simulink library "halin"  (R2021b)
settings: Solver=VariableStepAuto  StartTime=0.0  StopTime=10.0  RelTol=1e-3
undefined symbols (not defined in the file): TRUE
libraries: FVT_lib x177, hcu_lib x55
(part 5 of 17)

== system halin/HAL_IN/CAN5 ==
  DT_CAN5_SG_TBOX1 : Inport
  DT_CAN5_SG_TBOX2 : Inport  Port=2
  DT_CAN5_SG_TBOX3 : Inport  Port=3
  TBOX1 : Subsystem
  TBOX2 : Subsystem
  TBOX3 : Subsystem
  UnitConverter{,2,4,8..10} (6 alike) : DataTypeConversion  OutDataTypeStr=uint8
  UnitConverter{1,6,11..27} (19 alike) : DataTypeConversion  OutDataTypeStr=single
  UnitConverter28 : DataTypeConversion  OutDataTypeStr=uint32
  UnitConverter29 : DataTypeConversion  OutDataTypeStr=uint32
  UnitConverter3 : DataTypeConversion  OutDataTypeStr=uint16
  UnitConverter5 : DataTypeConversion  OutDataTypeStr=boolean
  UnitConverter7 : DataTypeConversion  OutDataTypeStr=boolean
  VHAL_CANMsgInvalidTBOX1_flg : Subsystem  AncestorBlock=FVT_lib/hal/MsgTimeoutJudge_CAN_AUTOSAR
      mask help: MeasumentTrigerEvent
      mask Display: fprintf('MsgTimeoutJudge_CAN\nAUTOSAR');
  VHAL_CANMsgInvalidTBOX2_flg : Subsystem  AncestorBlock=FVT_lib/hal/MsgTimeoutJudge_CAN_AUTOSAR
      mask help: MeasumentTrigerEvent
      mask Display: fprintf('MsgTimeoutJudge_CAN\nAUTOSAR');
  VHAL_CANMsgInvalidTBOX3_flg : Subsystem  AncestorBlock=FVT_lib/hal/MsgTimeoutJudge_CAN_AUTOSAR
      mask help: MeasumentTrigerEvent
      mask Display: fprintf('MsgTimeoutJudge_CAN\nAUTOSAR');
  bus_creator : BusCreator  Inputs=33
  HAL_CAN5_outputs : Outport
  wires:
  DT_CAN5_SG_TBOX1/1 -> [DT_CAN5_SG_TBOX1]
  DT_CAN5_SG_TBOX2/1 -> [DT_CAN5_SG_TBOX2]
  DT_CAN5_SG_TBOX3/1 -> [DT_CAN5_SG_TBOX3]
  [DT_CAN5_SG_TBOX1] -> TBOX1/1(DT_CAN5_SG_TBOX1)
  [DT_CAN5_SG_TBOX2] -> TBOX2/1(DT_CAN5_SG_TBOX2)
  [DT_CAN5_SG_TBOX3] -> TBOX3/1(DT_CAN5_SG_TBOX3)
  bus_creator/1 -> HAL_CAN5_outputs/1
  VHAL_CANMsgInvalidTBOX1_flg/1(Out) -> bus_creator/1
  TBOX1/1(VHAL_CbnPreACEnaReq_enum) -> [VHAL_CbnPreACEnaReq_enum]
  UnitConverter/1 -> bus_creator/2  "VHAL_CbnPreACEnaReq_enum"
  [VHAL_CbnPreACEnaReq_enum] -> UnitConverter/1
  TBOX1/2(VHAL_PowerOffTSet_cnt) -> [VHAL_PowerOffTSet_cnt]
  UnitConverter1/1 -> bus_creator/3  "VHAL_PowerOffTSet_cnt"
  [VHAL_PowerOffTSet_cnt] -> UnitConverter1/1
  TBOX1/3(VHAL_ReOutsideMirror_enum) -> [VHAL_ReOutsideMirror_enum]
  UnitConverter2/1 -> bus_creator/4  "VHAL_ReOutsideMirror_enum"
  [VHAL_ReOutsideMirror_enum] -> UnitConverter2/1
  TBOX1/4(VHAL_ReDoorLock_enum) -> [VHAL_ReDoorLock_enum]
  UnitConverter3/1 -> bus_creator/5  "VHAL_ReDoorLock_enum"
  [VHAL_ReDoorLock_enum] -> UnitConverter3/1
  TBOX1/5(VHAL_RePwrReqTbox_enum) -> [VHAL_RePwrReqTbox_enum]
  UnitConverter4/1 -> bus_creator/6  "VHAL_RePwrReqTbox_enum"
  [VHAL_RePwrReqTbox_enum] -> UnitConverter4/1
  TBOX1/6(VHAL_ReRadio_flg) -> [VHAL_ReRadio_flg]
  UnitConverter5/1 -> bus_creator/7  "VHAL_ReRadio_flg"
  [VHAL_ReRadio_flg] -> UnitConverter5/1
  TBOX1/7(VHAL_RemoteACTemp_C) -> [VHAL_RemoteACTemp_C]
  UnitConverter6/1 -> bus_creator/8  "VHAL_RemoteACTemp_C"
  [VHAL_RemoteACTemp_C] -> UnitConverter6/1
  TBOX1/8(VHAL_RemoteAutoReq_flg) -> [VHAL_RemoteAutoReq_flg]
  UnitConverter7/1 -> bus_creator/9  "VHAL_RemoteAutoReq_flg"
  [VHAL_RemoteAutoReq_flg] -> UnitConverter7/1
  TBOX1/9(VHAL_TBOXNETSIGSTR_enum) -> [VHAL_TBOXNETSIGSTR_enum]
  UnitConverter8/1 -> bus_creator/10  "VHAL_TBOXNETSIGSTR_enum"
  [VHAL_TBOXNETSIGSTR_enum] -> UnitConverter8/1
  TBOX1/10(VHAL_TBOXRemotePW_enum) -> [VHAL_TBOXRemotePW_enum]
  UnitConverter9/1 -> bus_creator/11  "VHAL_TBOXRemotePW_enum"
  [VHAL_TBOXRemotePW_enum] -> UnitConverter9/1
  TBOX1/11(VHAL_TBOXTESTSTATUS_enum) -> [VHAL_TBOXTESTSTATUS_enum]
  UnitConverter10/1 -> bus_creator/12  "VHAL_TBOXTESTSTATUS_enum"
  [VHAL_TBOXTESTSTATUS_enum] -> UnitConverter10/1
  VHAL_CANMsgInvalidTBOX2_flg/1(Out) -> bus_creator/13
  TBOX2/1(VHAL_TimeSyncFromBSDay_DAY) -> [VHAL_TimeSyncFromBSDay_DAY]
  UnitConverter11/1 -> bus_creator/14  "VHAL_TimeSyncFromBSDay_DAY"
  [VHAL_TimeSyncFromBSDay_DAY] -> UnitConverter11/1
  TBOX2/2(VHAL_TimeSyncFromBSHour_hr) -> [VHAL_TimeSyncFromBSHour_hr]
  UnitConverter12/1 -> bus_creator/15  "VHAL_TimeSyncFromBSHour_hr"
  [VHAL_TimeSyncFromBSHour_hr] -> UnitConverter12/1
  TBOX2/3(VHAL_TimeSyncFromBSMinute_min) -> [VHAL_TimeSyncFromBSMinute_min]
  UnitConverter13/1 -> bus_creator/16  "VHAL_TimeSyncFromBSMinute_min"
  [VHAL_TimeSyncFromBSMinute_min] -> UnitConverter13/1
  TBOX2/4(VHAL_TimeSyncFromBSMonth_MONTH) -> [VHAL_TimeSyncFromBSMonth_MONTH]
  UnitConverter14/1 -> bus_creator/17  "VHAL_TimeSyncFromBSMonth_MONTH"
  [VHAL_TimeSyncFromBSMonth_MONTH] -> UnitConverter14/1
  TBOX2/5(VHAL_TimeSyncFromBSSecond_s) -> [VHAL_TimeSyncFromBSSecond_s]
  UnitConverter15/1 -> bus_creator/18  "VHAL_TimeSyncFromBSSecond_s"
  [VHAL_TimeSyncFromBSSecond_s] -> UnitConverter15/1
  TBOX2/6(VHAL_TimeSyncFromBSYear_YEAR) -> [VHAL_TimeSyncFromBSYear_YEAR]
  UnitConverter16/1 -> bus_creator/19  "VHAL_TimeSyncFromBSYear_YEAR"
  [VHAL_TimeSyncFromBSYear_YEAR] -> UnitConverter16/1
  VHAL_CANMsgInvalidTBOX3_flg/1(Out) -> bus_creator/20
  TBOX3/1(VHAL_ChargePercentSet_pct) -> [VHAL_ChargePercentSet_pct]
  UnitConverter17/1 -> bus_creator/21  "VHAL_ChargePercentSet_pct"
  [VHAL_ChargePercentSet_pct] -> UnitConverter17/1
  TBOX3/2(VHAL_ReserveChargeOFFDay_DAY) -> [VHAL_ReserveChargeOFFDay_DAY]
  UnitConverter18/1 -> bus_creator/22  "VHAL_ReserveChargeOFFDay_DAY"
  [VHAL_ReserveChargeOFFDay_DAY] -> UnitConverter18/1
  TBOX3/3(VHAL_ReserveChargeOFFHour_hr) -> [VHAL_ReserveChargeOFFHour_hr]
  UnitConverter19/1 -> bus_creator/23  "VHAL_ReserveChargeOFFHour_hr"
  [VHAL_ReserveChargeOFFHour_hr] -> UnitConverter19/1
  TBOX3/4(VHAL_ReserveChargeOFFMinute_min) -> [VHAL_ReserveChargeOFFMinute_min]
  UnitConverter20/1 -> bus_creator/24  "VHAL_ReserveChargeOFFMinute_min"
  [VHAL_ReserveChargeOFFMinute_min] -> UnitConverter20/1
  TBOX3/5(VHAL_ReserveChargeOFFMonth_MONTH) -> [VHAL_ReserveChargeOFFMonth_MONTH]
  UnitConverter21/1 -> bus_creator/25  "VHAL_ReserveChargeOFFMonth_MONTH"
  [VHAL_ReserveChargeOFFMonth_MONTH] -> UnitConverter21/1
  TBOX3/6(VHAL_ReserveChargeOFFYear_YEAR) -> [VHAL_ReserveChargeOFFYear_YEAR]
  UnitConverter22/1 -> bus_creator/26  "VHAL_ReserveChargeOFFYear_YEAR"
  [VHAL_ReserveChargeOFFYear_YEAR] -> UnitConverter22/1
  TBOX3/7(VHAL_ReserveChargeOnDay_DAY) -> [VHAL_ReserveChargeOnDay_DAY]
  UnitConverter23/1 -> bus_creator/27  "VHAL_ReserveChargeOnDay_DAY"
  [VHAL_ReserveChargeOnDay_DAY] -> UnitConverter23/1
  TBOX3/8(VHAL_ReserveChargeOnHour_hr) -> [VHAL_ReserveChargeOnHour_hr]
  UnitConverter24/1 -> bus_creator/28  "VHAL_ReserveChargeOnHour_hr"
  [VHAL_ReserveChargeOnHour_hr] -> UnitConverter24/1
  TBOX3/9(VHAL_ReserveChargeOnMinute_min) -> [VHAL_ReserveChargeOnMinute_min]
  UnitConverter25/1 -> bus_creator/29  "VHAL_ReserveChargeOnMinute_min"
  [VHAL_ReserveChargeOnMinute_min] -> UnitConverter25/1
  TBOX3/10(VHAL_ReserveChargeOnMonth_MONTH) -> [VHAL_ReserveChargeOnMonth_MONTH]
  UnitConverter26/1 -> bus_creator/30  "VHAL_ReserveChargeOnMonth_MONTH"
  [VHAL_ReserveChargeOnMonth_MONTH] -> UnitConverter26/1
  TBOX3/11(VHAL_ReserveChargeOnYear_YEAR) -> [VHAL_ReserveChargeOnYear_YEAR]
  UnitConverter27/1 -> bus_creator/31  "VHAL_ReserveChargeOnYear_YEAR"
  [VHAL_ReserveChargeOnYear_YEAR] -> UnitConverter27/1
  TBOX3/12(VHAL_TBOXHWVER_enum) -> [VHAL_TBOXHWVER_enum]
  UnitConverter28/1 -> bus_creator/32  "VHAL_TBOXHWVER_enum"
  [VHAL_TBOXHWVER_enum] -> UnitConverter28/1
  TBOX3/13(VHAL_TBOXSWVER_enum) -> [VHAL_TBOXSWVER_enum]
  UnitConverter29/1 -> bus_creator/33  "VHAL_TBOXSWVER_enum"
  [VHAL_TBOXSWVER_enum] -> UnitConverter29/1

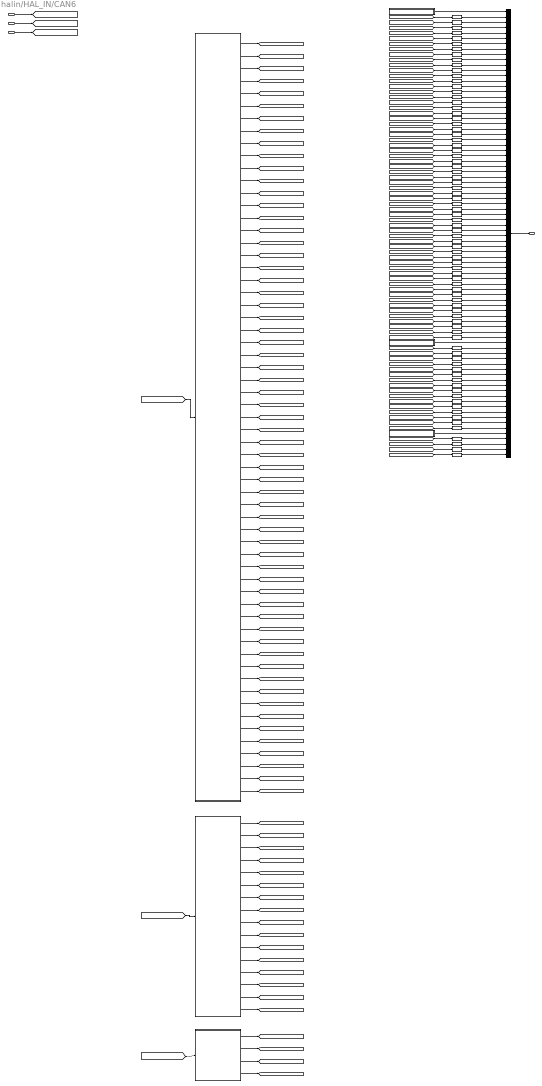
== system halin/HAL_IN/CAN6 ==
  DT_CAN6_SG_FCM1 : Inport
  DT_CAN6_SG_FCM3 : Inport  Port=2
  DT_CAN6_SG_SRR1 : Inport  Port=3
  FCM1 : Subsystem
  FCM3 : Subsystem
  SRR1 : Subsystem
  UnitConverter{,1..4,6..7,29..30,44,61..76} (26 alike) : DataTypeConversion  OutDataTypeStr=single
  UnitConverter{5,10..14,16,20,22..28,31..35,37..38,41..43,45,47,49,55,59..60,77..80} (35 alike) : DataTypeConversion  OutDataTypeStr=uint8
  UnitConverter{8..9,15,17..19,21,36,39..40,46,48,50..54,56..58} (20 alike) : DataTypeConversion  OutDataTypeStr=boolean
  VHAL_CANMsgInvalidFCM1_flg : Subsystem  AncestorBlock=FVT_lib/hal/MsgTimeoutJudge_CAN_AUTOSAR
      mask help: MeasumentTrigerEvent
      mask Display: fprintf('MsgTimeoutJudge_CAN\nAUTOSAR');
  VHAL_CANMsgInvalidFCM3_flg : Subsystem  AncestorBlock=FVT_lib/hal/MsgTimeoutJudge_CAN_AUTOSAR
      mask help: MeasumentTrigerEvent
      mask Display: fprintf('MsgTimeoutJudge_CAN\nAUTOSAR');
  VHAL_CANMsgInvalidSRR1_flg : Subsystem  AncestorBlock=FVT_lib/hal/MsgTimeoutJudge_CAN_AUTOSAR
      mask help: MeasumentTrigerEvent
      mask Display: fprintf('MsgTimeoutJudge_CAN\nAUTOSAR');
  bus_creator : BusCreator  Inputs=84
  HAL_CAN6_outputs : Outport
  wires:
  DT_CAN6_SG_FCM1/1 -> [DT_CAN6_SG_FCM1]
  DT_CAN6_SG_FCM3/1 -> [DT_CAN6_SG_FCM3]
  DT_CAN6_SG_SRR1/1 -> [DT_CAN6_SG_SRR1]
  [DT_CAN6_SG_FCM1] -> FCM1/1(DT_CAN6_SG_FCM1)
  [DT_CAN6_SG_FCM3] -> FCM3/1(DT_CAN6_SG_FCM3)
  [DT_CAN6_SG_SRR1] -> SRR1/1(DT_CAN6_SG_SRR1)
  bus_creator/1 -> HAL_CAN6_outputs/1
  VHAL_CANMsgInvalidFCM1_flg/1(Out) -> bus_creator/1
  FCM1/1(VHAL_ACCComfortBandLower_mps2) -> [VHAL_ACCComfortBandLower_mps2]
  UnitConverter/1 -> bus_creator/2  "VHAL_ACCComfortBandLower_mps2"
  [VHAL_ACCComfortBandLower_mps2] -> UnitConverter/1
  FCM1/2(VHAL_ACCComfortBandUpper_mps2) -> [VHAL_ACCComfortBandUpper_mps2]
  UnitConverter1/1 -> bus_creator/3  "VHAL_ACCComfortBandUpper_mps2"
  [VHAL_ACCComfortBandUpper_mps2] -> UnitConverter1/1
  FCM1/3(VHAL_ACCJerkLowerLimit_mps3) -> [VHAL_ACCJerkLowerLimit_mps3]
  UnitConverter2/1 -> bus_creator/4  "VHAL_ACCJerkLowerLimit_mps3"
  [VHAL_ACCJerkLowerLimit_mps3] -> UnitConverter2/1
  FCM1/4(VHAL_ACCJerkUpperLimit_mps3) -> [VHAL_ACCJerkUpperLimit_mps3]
  UnitConverter3/1 -> bus_creator/5  "VHAL_ACCJerkUpperLimit_mps3"
  [VHAL_ACCJerkUpperLimit_mps3] -> UnitConverter3/1
  FCM1/5(VHAL_ACCObjDist_m) -> [VHAL_ACCObjDist_m]
  UnitConverter4/1 -> bus_creator/6  "VHAL_ACCObjDist_m"
  [VHAL_ACCObjDist_m] -> UnitConverter4/1
  FCM1/6(VHAL_ACCObjDstLvl_enum) -> [VHAL_ACCObjDstLvl_enum]
  UnitConverter5/1 -> bus_creator/7  "VHAL_ACCObjDstLvl_enum"
  [VHAL_ACCObjDstLvl_enum] -> UnitConverter5/1
  FCM1/7(VHAL_ACCObjRelSpd_mps) -> [VHAL_ACCObjRelSpd_mps]
  UnitConverter6/1 -> bus_creator/8  "VHAL_ACCObjRelSpd_mps"
  [VHAL_ACCObjRelSpd_mps] -> UnitConverter6/1
  FCM1/8(VHAL_ACCRequiredAccel_mps2) -> [VHAL_ACCRequiredAccel_mps2]
  UnitConverter7/1 -> bus_creator/9  "VHAL_ACCRequiredAccel_mps2"
  [VHAL_ACCRequiredAccel_mps2] -> UnitConverter7/1
  FCM1/9(VHAL_ACCTakeoverReq_flg) -> [VHAL_ACCTakeoverReq_flg]
  UnitConverter8/1 -> bus_creator/10  "VHAL_ACCTakeoverReq_flg"
  [VHAL_ACCTakeoverReq_flg] -> UnitConverter8/1
  FCM1/10(VHAL_ACCVehHoldReq_flg) -> [VHAL_ACCVehHoldReq_flg]
  UnitConverter9/1 -> bus_creator/11  "VHAL_ACCVehHoldReq_flg"
  [VHAL_ACCVehHoldReq_flg] -> UnitConverter9/1
  FCM1/11(VHAL_ADASACCSta_enum) -> [VHAL_ADASACCSta_enum]
  UnitConverter10/1 -> bus_creator/12  "VHAL_ADASACCSta_enum"
  [VHAL_ADASACCSta_enum] -> UnitConverter10/1
  FCM1/12(VHAL_ADASAEBReq_enum) -> [VHAL_ADASAEBReq_enum]
  UnitConverter11/1 -> bus_creator/13  "VHAL_ADASAEBReq_enum"
  [VHAL_ADASAEBReq_enum] -> UnitConverter11/1
  FCM1/13(VHAL_ADASAEBSta_enum) -> [VHAL_ADASAEBSta_enum]
  UnitConverter12/1 -> bus_creator/14  "VHAL_ADASAEBSta_enum"
  [VHAL_ADASAEBSta_enum] -> UnitConverter12/1
  FCM1/14(VHAL_ADASCAMSpdLim_enum) -> [VHAL_ADASCAMSpdLim_enum]
  UnitConverter13/1 -> bus_creator/15  "VHAL_ADASCAMSpdLim_enum"
  [VHAL_ADASCAMSpdLim_enum] -> UnitConverter13/1
  FCM1/15(VHAL_ADASDBSReq_enum) -> [VHAL_ADASDBSReq_enum]
  UnitConverter14/1 -> bus_creator/16  "VHAL_ADASDBSReq_enum"
  [VHAL_ADASDBSReq_enum] -> UnitConverter14/1
  FCM1/16(VHAL_ADASFCWMute_flg) -> [VHAL_ADASFCWMute_flg]
  UnitConverter15/1 -> bus_creator/17  "VHAL_ADASFCWMute_flg"
  [VHAL_ADASFCWMute_flg] -> UnitConverter15/1
  FCM1/17(VHAL_ADASFCWSta_enum) -> [VHAL_ADASFCWSta_enum]
  UnitConverter16/1 -> bus_creator/18  "VHAL_ADASFCWSta_enum"
  [VHAL_ADASFCWSta_enum] -> UnitConverter16/1
  FCM1/18(VHAL_ADASFaultSta_flg) -> [VHAL_ADASFaultSta_flg]
  UnitConverter17/1 -> bus_creator/19  "VHAL_ADASFaultSta_flg"
  [VHAL_ADASFaultSta_flg] -> UnitConverter17/1
  FCM1/19(VHAL_ADASFltWrnReq_flg) -> [VHAL_ADASFltWrnReq_flg]
  UnitConverter18/1 -> bus_creator/20  "VHAL_ADASFltWrnReq_flg"
  [VHAL_ADASFltWrnReq_flg] -> UnitConverter18/1
  FCM1/20(VHAL_ADASForceIdle_flg) -> [VHAL_ADASForceIdle_flg]
  UnitConverter19/1 -> bus_creator/21  "VHAL_ADASForceIdle_flg"
  [VHAL_ADASForceIdle_flg] -> UnitConverter19/1
  FCM1/21(VHAL_ADASISASta_enum) -> [VHAL_ADASISASta_enum]
  UnitConverter20/1 -> bus_creator/22  "VHAL_ADASISASta_enum"
  [VHAL_ADASISASta_enum] -> UnitConverter20/1
  FCM1/22(VHAL_ADASLDWMute_flg) -> [VHAL_ADASLDWMute_flg]
  UnitConverter21/1 -> bus_creator/23  "VHAL_ADASLDWMute_flg"
  [VHAL_ADASLDWMute_flg] -> UnitConverter21/1
  FCM1/23(VHAL_ADASLDWSta_enum) -> [VHAL_ADASLDWSta_enum]
  UnitConverter22/1 -> bus_creator/24  "VHAL_ADASLDWSta_enum"
  [VHAL_ADASLDWSta_enum] -> UnitConverter22/1
  FCM1/24(VHAL_ADASLFCHandsOffWarning_enum) -> [VHAL_ADASLFCHandsOffWarning_enum]
  UnitConverter23/1 -> bus_creator/25  "VHAL_ADASLFCHandsOffWarning_enum"
  [VHAL_ADASLFCHandsOffWarning_enum] -> UnitConverter23/1
  FCM1/25(VHAL_ADASLFCSta_enum) -> [VHAL_ADASLFCSta_enum]
  UnitConverter24/1 -> bus_creator/26  "VHAL_ADASLFCSta_enum"
  [VHAL_ADASLFCSta_enum] -> UnitConverter24/1
  FCM1/26(VHAL_ADASLFCWarnSound_enum) -> [VHAL_ADASLFCWarnSound_enum]
  UnitConverter25/1 -> bus_creator/27  "VHAL_ADASLFCWarnSound_enum"
  [VHAL_ADASLFCWarnSound_enum] -> UnitConverter25/1
  FCM1/27(VHAL_ADASLKASta_enum) -> [VHAL_ADASLKASta_enum]
  UnitConverter26/1 -> bus_creator/28  "VHAL_ADASLKASta_enum"
  [VHAL_ADASLKASta_enum] -> UnitConverter26/1
  FCM1/28(VHAL_ADASLaneModeL_enum) -> [VHAL_ADASLaneModeL_enum]
  UnitConverter27/1 -> bus_creator/29  "VHAL_ADASLaneModeL_enum"
  [VHAL_ADASLaneModeL_enum] -> UnitConverter27/1
  FCM1/29(VHAL_ADASLaneModeR_enum) -> [VHAL_ADASLaneModeR_enum]
  UnitConverter28/1 -> bus_creator/30  "VHAL_ADASLaneModeR_enum"
  [VHAL_ADASLaneModeR_enum] -> UnitConverter28/1
  FCM1/30(VHAL_ADASLanecurveL_raw32) -> [VHAL_ADASLanecurveL_raw32]
  UnitConverter29/1 -> bus_creator/31  "VHAL_ADASLanecurveL_raw32"
  [VHAL_ADASLanecurveL_raw32] -> UnitConverter29/1
  FCM1/31(VHAL_ADASLanecurveR_raw32) -> [VHAL_ADASLanecurveR_raw32]
  UnitConverter30/1 -> bus_creator/32  "VHAL_ADASLanecurveR_raw32"
  [VHAL_ADASLanecurveR_raw32] -> UnitConverter30/1
  FCM1/32(VHAL_ADASLanetypeL_enum) -> [VHAL_ADASLanetypeL_enum]
  UnitConverter31/1 -> bus_creator/33  "VHAL_ADASLanetypeL_enum"
  [VHAL_ADASLanetypeL_enum] -> UnitConverter31/1
  FCM1/33(VHAL_ADASLanetypeR_enum) -> [VHAL_ADASLanetypeR_enum]
  UnitConverter32/1 -> bus_creator/34  "VHAL_ADASLanetypeR_enum"
  [VHAL_ADASLanetypeR_enum] -> UnitConverter32/1
  FCM1/34(VHAL_ADASSLIFSpdLim_enum) -> [VHAL_ADASSLIFSpdLim_enum]
  UnitConverter33/1 -> bus_creator/35  "VHAL_ADASSLIFSpdLim_enum"
  [VHAL_ADASSLIFSpdLim_enum] -> UnitConverter33/1
  FCM1/35(VHAL_ADASSLIFSta_enum) -> [VHAL_ADASSLIFSta_enum]
  UnitConverter34/1 -> bus_creator/36  "VHAL_ADASSLIFSta_enum"
  [VHAL_ADASSLIFSta_enum] -> UnitConverter34/1
  FCM1/36(VHAL_ADASShftPosnReq_enum) -> [VHAL_ADASShftPosnReq_enum]
  UnitConverter35/1 -> bus_creator/37  "VHAL_ADASShftPosnReq_enum"
  [VHAL_ADASShftPosnReq_enum] -> UnitConverter35/1
  FCM1/37(VHAL_ADASShftPosnReqA_flg) -> [VHAL_ADASShftPosnReqA_flg]
  UnitConverter36/1 -> bus_creator/38  "VHAL_ADASShftPosnReqA_flg"
  [VHAL_ADASShftPosnReqA_flg] -> UnitConverter36/1
  FCM1/38(VHAL_ADASVehSpdLim_enum) -> [VHAL_ADASVehSpdLim_enum]
  UnitConverter37/1 -> bus_creator/39  "VHAL_ADASVehSpdLim_enum"
  [VHAL_ADASVehSpdLim_enum] -> UnitConverter37/1
  FCM1/39(VHAL_ADASWarningMsg_enum) -> [VHAL_ADASWarningMsg_enum]
  UnitConverter38/1 -> bus_creator/40  "VHAL_ADASWarningMsg_enum"
  [VHAL_ADASWarningMsg_enum] -> UnitConverter38/1
  FCM1/40(VHAL_AEBVehHoldReq_flg) -> [VHAL_AEBVehHoldReq_flg]
  UnitConverter39/1 -> bus_creator/41  "VHAL_AEBVehHoldReq_flg"
  [VHAL_AEBVehHoldReq_flg] -> UnitConverter39/1
  FCM1/41(VHAL_CameraBlockage_flg) -> [VHAL_CameraBlockage_flg]
  UnitConverter40/1 -> bus_creator/42  "VHAL_CameraBlockage_flg"
  [VHAL_CameraBlockage_flg] -> UnitConverter40/1
  FCM1/42(VHAL_FCM1Checksum_enum) -> [VHAL_FCM1Checksum_enum]
  UnitConverter41/1 -> bus_creator/43  "VHAL_FCM1Checksum_enum"
  [VHAL_FCM1Checksum_enum] -> UnitConverter41/1
  FCM1/43(VHAL_FCM1LifeCount_enum) -> [VHAL_FCM1LifeCount_enum]
  UnitConverter42/1 -> bus_creator/44  "VHAL_FCM1LifeCount_enum"
  [VHAL_FCM1LifeCount_enum] -> UnitConverter42/1
  FCM1/44(VHAL_FCMACCmode_enum) -> [VHAL_FCMACCmode_enum]
  UnitConverter43/1 -> bus_creator/45  "VHAL_FCMACCmode_enum"
  [VHAL_FCMACCmode_enum] -> UnitConverter43/1
  FCM1/45(VHAL_FCMLKAStrToqReq_Nm) -> [VHAL_FCMLKAStrToqReq_Nm]
  UnitConverter44/1 -> bus_creator/46  "VHAL_FCMLKAStrToqReq_Nm"
  [VHAL_FCMLKAStrToqReq_Nm] -> UnitConverter44/1
  FCM1/46(VHAL_FCMLKATOIAct_enum) -> [VHAL_FCMLKATOIAct_enum]
  UnitConverter45/1 -> bus_creator/47  "VHAL_FCMLKATOIAct_enum"
  [VHAL_FCMLKATOIAct_enum] -> UnitConverter45/1
  FCM1/47(VHAL_FCMLKATOIFault_flg) -> [VHAL_FCMLKATOIFault_flg]
  UnitConverter46/1 -> bus_creator/48  "VHAL_FCMLKATOIFault_flg"
  [VHAL_FCMLKATOIFault_flg] -> UnitConverter46/1
  FCM1/48(VHAL_ForceLowBeam_enum) -> [VHAL_ForceLowBeam_enum]
  UnitConverter47/1 -> bus_creator/49  "VHAL_ForceLowBeam_enum"
  [VHAL_ForceLowBeam_enum] -> UnitConverter47/1
  FCM1/49(VHAL_HazardWarningReq_flg) -> [VHAL_HazardWarningReq_flg]
  UnitConverter48/1 -> bus_creator/50  "VHAL_HazardWarningReq_flg"
  [VHAL_HazardWarningReq_flg] -> UnitConverter48/1
  FCM1/50(VHAL_ISAWarningMsg_enum) -> [VHAL_ISAWarningMsg_enum]
  UnitConverter49/1 -> bus_creator/51  "VHAL_ISAWarningMsg_enum"
  [VHAL_ISAWarningMsg_enum] -> UnitConverter49/1
  FCM1/51(VHAL_LKAHODDisplayWarning_flg) -> [VHAL_LKAHODDisplayWarning_flg]
  UnitConverter50/1 -> bus_creator/52  "VHAL_LKAHODDisplayWarning_flg"
  [VHAL_LKAHODDisplayWarning_flg] -> UnitConverter50/1
  FCM1/52(VHAL_LKAHODSoundWarning_flg) -> [VHAL_LKAHODSoundWarning_flg]
  UnitConverter51/1 -> bus_creator/53  "VHAL_LKAHODSoundWarning_flg"
  [VHAL_LKAHODSoundWarning_flg] -> UnitConverter51/1
  FCM1/53(VHAL_LVDAACCStatusInformation_flg) -> [VHAL_LVDAACCStatusInformation_flg]
  UnitConverter52/1 -> bus_creator/54  "VHAL_LVDAACCStatusInformation_flg"
  [VHAL_LVDAACCStatusInformation_flg] -> UnitConverter52/1
  FCM1/54(VHAL_LVDADisabled_flg) -> [VHAL_LVDADisabled_flg]
  UnitConverter53/1 -> bus_creator/55  "VHAL_LVDADisabled_flg"
  [VHAL_LVDADisabled_flg] -> UnitConverter53/1
  FCM1/55(VHAL_LVDAFailinfo_flg) -> [VHAL_LVDAFailinfo_flg]
  UnitConverter54/1 -> bus_creator/56  "VHAL_LVDAFailinfo_flg"
  [VHAL_LVDAFailinfo_flg] -> UnitConverter54/1
  FCM1/56(VHAL_LVDAMuteSta_enum) -> [VHAL_LVDAMuteSta_enum]
  UnitConverter55/1 -> bus_creator/57  "VHAL_LVDAMuteSta_enum"
  [VHAL_LVDAMuteSta_enum] -> UnitConverter55/1
  FCM1/57(VHAL_LVDAWarning_flg) -> [VHAL_LVDAWarning_flg]
  UnitConverter56/1 -> bus_creator/58  "VHAL_LVDAWarning_flg"
  [VHAL_LVDAWarning_flg] -> UnitConverter56/1
  FCM1/58(VHAL_LeftTurnLightReq_flg) -> [VHAL_LeftTurnLightReq_flg]
  UnitConverter57/1 -> bus_creator/59  "VHAL_LeftTurnLightReq_flg"
  [VHAL_LeftTurnLightReq_flg] -> UnitConverter57/1
  FCM1/59(VHAL_RightTurnLightReq_flg) -> [VHAL_RightTurnLightReq_flg]
  UnitConverter58/1 -> bus_creator/60  "VHAL_RightTurnLightReq_flg"
  [VHAL_RightTurnLightReq_flg] -> UnitConverter58/1
  FCM1/60(VHAL_TargetType_enum) -> [VHAL_TargetType_enum]
  UnitConverter59/1 -> bus_creator/61  "VHAL_TargetType_enum"
  [VHAL_TargetType_enum] -> UnitConverter59/1
  FCM1/61(VHAL_TimeGapLevel_enum) -> [VHAL_TimeGapLevel_enum]
  UnitConverter60/1 -> bus_creator/62  "VHAL_TimeGapLevel_enum"
  [VHAL_TimeGapLevel_enum] -> UnitConverter60/1
  VHAL_CANMsgInvalidFCM3_flg/1(Out) -> bus_creator/63
  FCM3/1(VHAL_MELaneCurvDervLt_raw32) -> [VHAL_MELaneCurvDervLt_raw32]
  UnitConverter61/1 -> bus_creator/64  "VHAL_MELaneCurvDervLt_raw32"
  [VHAL_MELaneCurvDervLt_raw32] -> UnitConverter61/1
  FCM3/2(VHAL_MELaneCurvDervLt2_raw32) -> [VHAL_MELaneCurvDervLt2_raw32]
  UnitConverter62/1 -> bus_creator/65  "VHAL_MELaneCurvDervLt2_raw32"
  [VHAL_MELaneCurvDervLt2_raw32] -> UnitConverter62/1
  FCM3/3(VHAL_MELaneCurvDervRt_raw32) -> [VHAL_MELaneCurvDervRt_raw32]
  UnitConverter63/1 -> bus_creator/66  "VHAL_MELaneCurvDervRt_raw32"
  [VHAL_MELaneCurvDervRt_raw32] -> UnitConverter63/1
  FCM3/4(VHAL_MELaneCurvDervRt2_raw32) -> [VHAL_MELaneCurvDervRt2_raw32]
  UnitConverter64/1 -> bus_creator/67  "VHAL_MELaneCurvDervRt2_raw32"
  [VHAL_MELaneCurvDervRt2_raw32] -> UnitConverter64/1
  FCM3/5(VHAL_MELaneCurvLt_raw32) -> [VHAL_MELaneCurvLt_raw32]
  UnitConverter65/1 -> bus_creator/68  "VHAL_MELaneCurvLt_raw32"
  [VHAL_MELaneCurvLt_raw32] -> UnitConverter65/1
  FCM3/6(VHAL_MELaneCurvLt2_raw32) -> [VHAL_MELaneCurvLt2_raw32]
  UnitConverter66/1 -> bus_creator/69  "VHAL_MELaneCurvLt2_raw32"
  [VHAL_MELaneCurvLt2_raw32] -> UnitConverter66/1
  FCM3/7(VHAL_MELaneCurvRt_raw32) -> [VHAL_MELaneCurvRt_raw32]
  UnitConverter67/1 -> bus_creator/70  "VHAL_MELaneCurvRt_raw32"
  [VHAL_MELaneCurvRt_raw32] -> UnitConverter67/1
  FCM3/8(VHAL_MELaneCurvRt2_raw32) -> [VHAL_MELaneCurvRt2_raw32]
  UnitConverter68/1 -> bus_creator/71  "VHAL_MELaneCurvRt2_raw32"
  [VHAL_MELaneCurvRt2_raw32] -> UnitConverter68/1
  FCM3/9(VHAL_MELaneHeadAngLt_radians) -> [VHAL_MELaneHeadAngLt_radians]
  UnitConverter69/1 -> bus_creator/72  "VHAL_MELaneHeadAngLt_radians"
  [VHAL_MELaneHeadAngLt_radians] -> UnitConverter69/1
  FCM3/10(VHAL_MELaneHeadAngLt2_radians) -> [VHAL_MELaneHeadAngLt2_radians]
  UnitConverter70/1 -> bus_creator/73  "VHAL_MELaneHeadAngLt2_radians"
  [VHAL_MELaneHeadAngLt2_radians] -> UnitConverter70/1
  FCM3/11(VHAL_MELaneHeadAngRt_radians) -> [VHAL_MELaneHeadAngRt_radians]
  UnitConverter71/1 -> bus_creator/74  "VHAL_MELaneHeadAngRt_radians"
  [VHAL_MELaneHeadAngRt_radians] -> UnitConverter71/1
  FCM3/12(VHAL_MELaneHeadAngRt2_radians) -> [VHAL_MELaneHeadAngRt2_radians]
  UnitConverter72/1 -> bus_creator/75  "VHAL_MELaneHeadAngRt2_radians"
  [VHAL_MELaneHeadAngRt2_radians] -> UnitConverter72/1
  FCM3/13(VHAL_MELanePosLt_m) -> [VHAL_MELanePosLt_m]
  UnitConverter73/1 -> bus_creator/76  "VHAL_MELanePosLt_m"
  [VHAL_MELanePosLt_m] -> UnitConverter73/1
  FCM3/14(VHAL_MELanePosLt2_m) -> [VHAL_MELanePosLt2_m]
  UnitConverter74/1 -> bus_creator/77  "VHAL_MELanePosLt2_m"
  [VHAL_MELanePosLt2_m] -> UnitConverter74/1
  FCM3/15(VHAL_MELanePosRt_m) -> [VHAL_MELanePosRt_m]
  UnitConverter75/1 -> bus_creator/78  "VHAL_MELanePosRt_m"
  [VHAL_MELanePosRt_m] -> UnitConverter75/1
  FCM3/16(VHAL_MELanePosRt2_m) -> [VHAL_MELanePosRt2_m]
  UnitConverter76/1 -> bus_creator/79  "VHAL_MELanePosRt2_m"
  [VHAL_MELanePosRt2_m] -> UnitConverter76/1
  VHAL_CANMsgInvalidSRR1_flg/1(Out) -> bus_creator/80
  SRR1/1(VHAL_SRRBSDWarnL_enum) -> [VHAL_SRRBSDWarnL_enum]
  UnitConverter77/1 -> bus_creator/81  "VHAL_SRRBSDWarnL_enum"
  [VHAL_SRRBSDWarnL_enum] -> UnitConverter77/1
  SRR1/2(VHAL_SRRBSDWarnR_enum) -> [VHAL_SRRBSDWarnR_enum]
  UnitConverter78/1 -> bus_creator/82  "VHAL_SRRBSDWarnR_enum"
  [VHAL_SRRBSDWarnR_enum] -> UnitConverter78/1
  SRR1/3(VHAL_SRRODAWarnL_enum) -> [VHAL_SRRODAWarnL_enum]
  UnitConverter79/1 -> bus_creator/83  "VHAL_SRRODAWarnL_enum"
  [VHAL_SRRODAWarnL_enum] -> UnitConverter79/1
  SRR1/4(VHAL_SRRODAWarnR_enum) -> [VHAL_SRRODAWarnR_enum]
  UnitConverter80/1 -> bus_creator/84  "VHAL_SRRODAWarnR_enum"
  [VHAL_SRRODAWarnR_enum] -> UnitConverter80/1

== system halin/HAL_IN/CAN1/ABM1 ==
  DT_CAN1_SG_ABM1 : Inport
  ABMPassengerODSSta : Subsystem
  ABMRearPassengerCTRODSSta : Subsystem
  ABMRearPassengerLHODSSta : Subsystem
  ABMRearPassengerRHODSSta : Subsystem
  AirBagFailCmd : Subsystem
  ChecksumABM1 : Subsystem
  CrashOutputSts : Subsystem
  DriverSeatBeltCmd : Subsystem
  LifeCountABM1 : Subsystem
  PABSwitchCmd : Subsystem
  PsngrSeatBeltCmd : Subsystem
  RCenterSeatBeltCmd : Subsystem
  RDriverSeatBeltCmd : Subsystem
  RPsngrSeatBeltCmd : Subsystem
  TLHPsngrSeatBeltCmd : Subsystem
  TRHPsngrSeatBeltCmd : Subsystem
  bus_selector : BusSelector  OutputSignals=CAN1_ABM_Passenger_ODS_Sta
  bus_selector1 : BusSelector  OutputSignals=CAN1_ABM_RearPassengerCTR_ODS_Sta
  bus_selector10 : BusSelector  OutputSignals=CAN1_PsngrSeatBeltCmd
  bus_selector11 : BusSelector  OutputSignals=CAN1_RCenterSeatBeltCmd
  bus_selector12 : BusSelector  OutputSignals=CAN1_RDriverSeatBeltCmd
  bus_selector13 : BusSelector  OutputSignals=CAN1_RPsngrSeatBeltCmd
  bus_selector14 : BusSelector  OutputSignals=CAN1_TLHPsngrSeatBeltCmd
  bus_selector15 : BusSelector  OutputSignals=CAN1_TRHPsngrSeatBeltCmd
  bus_selector2 : BusSelector  OutputSignals=CAN1_ABM_RearPassengerLH_ODS_Sta
  bus_selector3 : BusSelector  OutputSignals=CAN1_ABM_RearPassengerRH_ODS_Sta
  bus_selector4 : BusSelector  OutputSignals=CAN1_AirBagFailCmd
  bus_selector5 : BusSelector  OutputSignals=CAN1_Checksum_ABM1
  bus_selector6 : BusSelector  OutputSignals=CAN1_CrashOutputSts
  bus_selector7 : BusSelector  OutputSignals=CAN1_DriverSeatBeltCmd
  bus_selector8 : BusSelector  OutputSignals=CAN1_LifeCount_ABM1
  bus_selector9 : BusSelector  OutputSignals=CAN1_PABSwitchCmd
  VHAL_ABMPassengerODSSta_flg : Outport
  VHAL_ABMRearPassengerCTRODSSta_flg : Outport  Port=2
  VHAL_ABMRearPassengerLHODSSta_flg : Outport  Port=3
  VHAL_ABMRearPassengerRHODSSta_flg : Outport  Port=4
  VHAL_AirBagFailCmd_flg : Outport  Port=5
  VHAL_ChecksumABM1_enum : Outport  Port=6
  VHAL_CrashOutputSts_enum : Outport  Port=7
  VHAL_DriverSeatBeltCmd_flg : Outport  Port=8
  VHAL_LifeCountABM1_enum : Outport  Port=9
  VHAL_PABSwitchCmd_flg : Outport  Port=10
  VHAL_PsngrSeatBeltCmd_flg : Outport  Port=11
  VHAL_RCenterSeatBeltCmd_flg : Outport  Port=12
  VHAL_RDriverSeatBeltCmd_flg : Outport  Port=13
  VHAL_RPsngrSeatBeltCmd_flg : Outport  Port=14
  VHAL_TLHPsngrSeatBeltCmd_flg : Outport  Port=15
  VHAL_TRHPsngrSeatBeltCmd_flg : Outport  Port=16
  wires:
  DT_CAN1_SG_ABM1/1 -> [DT_CAN1_SG_ABM1]
  [DT_CAN1_SG_ABM1] -> bus_selector/1
  bus_selector/1 -> ABMPassengerODSSta/1(ABM_Passenger_ODS_Sta)  "<CAN1_ABM_Passenger_ODS_Sta>"
  ABMPassengerODSSta/1(VHAL_ABMPassengerODSSta_flg) -> VHAL_ABMPassengerODSSta_flg/1
  [DT_CAN1_SG_ABM1] -> bus_selector1/1
  bus_selector1/1 -> ABMRearPassengerCTRODSSta/1(ABM_RearPassengerCTR_ODS_Sta)  "<CAN1_ABM_RearPassengerCTR_ODS_Sta>"
  ABMRearPassengerCTRODSSta/1(VHAL_ABMRearPassengerCTRODSSta_flg) -> VHAL_ABMRearPassengerCTRODSSta_flg/1
  [DT_CAN1_SG_ABM1] -> bus_selector2/1
  bus_selector2/1 -> ABMRearPassengerLHODSSta/1(ABM_RearPassengerLH_ODS_Sta)  "<CAN1_ABM_RearPassengerLH_ODS_Sta>"
  ABMRearPassengerLHODSSta/1(VHAL_ABMRearPassengerLHODSSta_flg) -> VHAL_ABMRearPassengerLHODSSta_flg/1
  [DT_CAN1_SG_ABM1] -> bus_selector3/1
  bus_selector3/1 -> ABMRearPassengerRHODSSta/1(ABM_RearPassengerRH_ODS_Sta)  "<CAN1_ABM_RearPassengerRH_ODS_Sta>"
  ABMRearPassengerRHODSSta/1(VHAL_ABMRearPassengerRHODSSta_flg) -> VHAL_ABMRearPassengerRHODSSta_flg/1
  [DT_CAN1_SG_ABM1] -> bus_selector4/1
  bus_selector4/1 -> AirBagFailCmd/1(AirBagFailCmd)  "<CAN1_AirBagFailCmd>"
  AirBagFailCmd/1(VHAL_AirBagFailCmd_flg) -> VHAL_AirBagFailCmd_flg/1
  [DT_CAN1_SG_ABM1] -> bus_selector5/1
  bus_selector5/1 -> ChecksumABM1/1(Checksum_ABM1)  "<CAN1_Checksum_ABM1>"
  ChecksumABM1/1(VHAL_ChecksumABM1_enum) -> VHAL_ChecksumABM1_enum/1
  [DT_CAN1_SG_ABM1] -> bus_selector6/1
  bus_selector6/1 -> CrashOutputSts/1(CrashOutputSts)  "<CAN1_CrashOutputSts>"
  CrashOutputSts/1(VHAL_CrashOutputSts_enum) -> VHAL_CrashOutputSts_enum/1
  [DT_CAN1_SG_ABM1] -> bus_selector7/1
  bus_selector7/1 -> DriverSeatBeltCmd/1(DriverSeatBeltCmd)  "<CAN1_DriverSeatBeltCmd>"
  DriverSeatBeltCmd/1(VHAL_DriverSeatBeltCmd_flg) -> VHAL_DriverSeatBeltCmd_flg/1
  [DT_CAN1_SG_ABM1] -> bus_selector8/1
  bus_selector8/1 -> LifeCountABM1/1(LifeCount_ABM1)  "<CAN1_LifeCount_ABM1>"
  LifeCountABM1/1(VHAL_LifeCountABM1_enum) -> VHAL_LifeCountABM1_enum/1
  [DT_CAN1_SG_ABM1] -> bus_selector9/1
  bus_selector9/1 -> PABSwitchCmd/1(PABSwitchCmd)  "<CAN1_PABSwitchCmd>"
  PABSwitchCmd/1(VHAL_PABSwitchCmd_flg) -> VHAL_PABSwitchCmd_flg/1
  [DT_CAN1_SG_ABM1] -> bus_selector10/1
  bus_selector10/1 -> PsngrSeatBeltCmd/1(PsngrSeatBeltCmd)  "<CAN1_PsngrSeatBeltCmd>"
  PsngrSeatBeltCmd/1(VHAL_PsngrSeatBeltCmd_flg) -> VHAL_PsngrSeatBeltCmd_flg/1
  [DT_CAN1_SG_ABM1] -> bus_selector11/1
  bus_selector11/1 -> RCenterSeatBeltCmd/1(RCenterSeatBeltCmd)  "<CAN1_RCenterSeatBeltCmd>"
  RCenterSeatBeltCmd/1(VHAL_RCenterSeatBeltCmd_flg) -> VHAL_RCenterSeatBeltCmd_flg/1
  [DT_CAN1_SG_ABM1] -> bus_selector12/1
  bus_selector12/1 -> RDriverSeatBeltCmd/1(RDriverSeatBeltCmd)  "<CAN1_RDriverSeatBeltCmd>"
  RDriverSeatBeltCmd/1(VHAL_RDriverSeatBeltCmd_flg) -> VHAL_RDriverSeatBeltCmd_flg/1
  [DT_CAN1_SG_ABM1] -> bus_selector13/1
  bus_selector13/1 -> RPsngrSeatBeltCmd/1(RPsngrSeatBeltCmd)  "<CAN1_RPsngrSeatBeltCmd>"
  RPsngrSeatBeltCmd/1(VHAL_RPsngrSeatBeltCmd_flg) -> VHAL_RPsngrSeatBeltCmd_flg/1
  [DT_CAN1_SG_ABM1] -> bus_selector14/1
  bus_selector14/1 -> TLHPsngrSeatBeltCmd/1(TLHPsngrSeatBeltCmd)  "<CAN1_TLHPsngrSeatBeltCmd>"
  TLHPsngrSeatBeltCmd/1(VHAL_TLHPsngrSeatBeltCmd_flg) -> VHAL_TLHPsngrSeatBeltCmd_flg/1
  [DT_CAN1_SG_ABM1] -> bus_selector15/1
  bus_selector15/1 -> TRHPsngrSeatBeltCmd/1(TRHPsngrSeatBeltCmd)  "<CAN1_TRHPsngrSeatBeltCmd>"
  TRHPsngrSeatBeltCmd/1(VHAL_TRHPsngrSeatBeltCmd_flg) -> VHAL_TRHPsngrSeatBeltCmd_flg/1

== system halin/HAL_IN/CAN1/EPB1 ==
  DT_CAN1_SG_EPB1 : Inport
  DOASta : Subsystem
  EPBCarWashMode : Subsystem
  EPBErrSta : Subsystem
  EPBExtApplyAvail : Subsystem
  EPBExtReleaseAvail : Subsystem
  EPBSta : Subsystem
  bus_selector : BusSelector  OutputSignals=CAN1_DOA_Sta
  bus_selector1 : BusSelector  OutputSignals=CAN1_EPBCarWashMode
  bus_selector2 : BusSelector  OutputSignals=CAN1_EPBErrSta
  bus_selector3 : BusSelector  OutputSignals=CAN1_EPBExtApplyAvail
  bus_selector4 : BusSelector  OutputSignals=CAN1_EPBExtReleaseAvail
  bus_selector5 : BusSelector  OutputSignals=CAN1_EPBSta
  VHAL_DOASta_flg : Outport
  VHAL_EPBCarWashMode_flg : Outport  Port=2
  VHAL_EPBErrSta_enum : Outport  Port=3
  VHAL_EPBExtApplyAvail_flg : Outport  Port=4
  VHAL_EPBExtReleaseAvail_flg : Outport  Port=5
  VHAL_EPBSta_enum : Outport  Port=6
  wires:
  DT_CAN1_SG_EPB1/1 -> [DT_CAN1_SG_EPB1]
  [DT_CAN1_SG_EPB1] -> bus_selector/1
  bus_selector/1 -> DOASta/1(DOA_Sta)  "<CAN1_DOA_Sta>"
  DOASta/1(VHAL_DOASta_flg) -> VHAL_DOASta_flg/1
  [DT_CAN1_SG_EPB1] -> bus_selector1/1
  bus_selector1/1 -> EPBCarWashMode/1(EPBCarWashMode)  "<CAN1_EPBCarWashMode>"
  EPBCarWashMode/1(VHAL_EPBCarWashMode_flg) -> VHAL_EPBCarWashMode_flg/1
  [DT_CAN1_SG_EPB1] -> bus_selector2/1
  bus_selector2/1 -> EPBErrSta/1(EPBErrSta)  "<CAN1_EPBErrSta>"
  EPBErrSta/1(VHAL_EPBErrSta_enum) -> VHAL_EPBErrSta_enum/1
  [DT_CAN1_SG_EPB1] -> bus_selector3/1
  bus_selector3/1 -> EPBExtApplyAvail/1(EPBExtApplyAvail)  "<CAN1_EPBExtApplyAvail>"
  EPBExtApplyAvail/1(VHAL_EPBExtApplyAvail_flg) -> VHAL_EPBExtApplyAvail_flg/1
  [DT_CAN1_SG_EPB1] -> bus_selector4/1
  bus_selector4/1 -> EPBExtReleaseAvail/1(EPBExtReleaseAvail)  "<CAN1_EPBExtReleaseAvail>"
  EPBExtReleaseAvail/1(VHAL_EPBExtReleaseAvail_flg) -> VHAL_EPBExtReleaseAvail_flg/1
  [DT_CAN1_SG_EPB1] -> bus_selector5/1
  bus_selector5/1 -> EPBSta/1(EPBSta)  "<CAN1_EPBSta>"
  EPBSta/1(VHAL_EPBSta_enum) -> VHAL_EPBSta_enum/1

== system halin/HAL_IN/CAN1/EPS1 ==
  DT_CAN1_SG_EPS1 : Inport
  DriIntend : Subsystem
  EPSAOIControl : Subsystem
  EpasFailed : Subsystem
  SASAngle : Subsystem
  SASCAL : Subsystem
  SASSpeed : Subsystem
  SASSpeedValid : Subsystem
  SASV : Subsystem
  bus_selector : BusSelector  OutputSignals=CAN1_DriIntend
  bus_selector1 : BusSelector  OutputSignals=CAN1_EPS_AOI_Control
  bus_selector2 : BusSelector  OutputSignals=CAN1_EpasFailed
  bus_selector3 : BusSelector  OutputSignals=CAN1_SAS_Angle
  bus_selector4 : BusSelector  OutputSignals=CAN1_SAS_CAL
  bus_selector5 : BusSelector  OutputSignals=CAN1_SAS_Speed
  bus_selector6 : BusSelector  OutputSignals=CAN1_SAS_Speed_Valid
  bus_selector7 : BusSelector  OutputSignals=CAN1_SAS_V
  VHAL_DriIntend_enum : Outport
  VHAL_EPSAOIControl_enum : Outport  Port=2
  VHAL_EpasFailed_enum : Outport  Port=3
  VHAL_SASAngle_Deg : Outport  Port=4
  VHAL_SASCAL_flg : Outport  Port=5
  VHAL_SASSpeed_degps : Outport  Port=6
  VHAL_SASSpeedValid_flg : Outport  Port=7
  VHAL_SASV_flg : Outport  Port=8
  wires:
  DT_CAN1_SG_EPS1/1 -> [DT_CAN1_SG_EPS1]
  [DT_CAN1_SG_EPS1] -> bus_selector/1
  bus_selector/1 -> DriIntend/1(DriIntend)  "<CAN1_DriIntend>"
  DriIntend/1(VHAL_DriIntend_enum) -> VHAL_DriIntend_enum/1
  [DT_CAN1_SG_EPS1] -> bus_selector1/1
  bus_selector1/1 -> EPSAOIControl/1(EPS_AOI_Control)  "<CAN1_EPS_AOI_Control>"
  EPSAOIControl/1(VHAL_EPSAOIControl_enum) -> VHAL_EPSAOIControl_enum/1
  [DT_CAN1_SG_EPS1] -> bus_selector2/1
  bus_selector2/1 -> EpasFailed/1(EpasFailed)  "<CAN1_EpasFailed>"
  EpasFailed/1(VHAL_EpasFailed_enum) -> VHAL_EpasFailed_enum/1
  [DT_CAN1_SG_EPS1] -> bus_selector3/1
  bus_selector3/1 -> SASAngle/1(SAS_Angle)  "<CAN1_SAS_Angle>"
  SASAngle/1(VHAL_SASAngle_Deg) -> VHAL_SASAngle_Deg/1
  [DT_CAN1_SG_EPS1] -> bus_selector4/1
  bus_selector4/1 -> SASCAL/1(SAS_CAL)  "<CAN1_SAS_CAL>"
  SASCAL/1(VHAL_SASCAL_flg) -> VHAL_SASCAL_flg/1
  [DT_CAN1_SG_EPS1] -> bus_selector5/1
  bus_selector5/1 -> SASSpeed/1(SAS_Speed)  "<CAN1_SAS_Speed>"
  SASSpeed/1(VHAL_SASSpeed_degps) -> VHAL_SASSpeed_degps/1
  [DT_CAN1_SG_EPS1] -> bus_selector6/1
  bus_selector6/1 -> SASSpeedValid/1(SAS_Speed_Valid)  "<CAN1_SAS_Speed_Valid>"
  SASSpeedValid/1(VHAL_SASSpeedValid_flg) -> VHAL_SASSpeedValid_flg/1
  [DT_CAN1_SG_EPS1] -> bus_selector7/1
  bus_selector7/1 -> SASV/1(SAS_V)  "<CAN1_SAS_V>"
  SASV/1(VHAL_SASV_flg) -> VHAL_SASV_flg/1
